simulink model "Three_phase_IM_PF_correction_Stardelta_Capacitor_Bank"  (R2024a)
settings: Solver=VariableStepAuto  StartTime=0.0  StopTime=2  RelTol=1e-3
libraries: spsRMSLib x10, spsSeriesRLCBranchLib x6, spsAsynchronousMachineSIUnitsLib x5, spsPower3phInstantaneousLib x5, spsThreePhaseVIMeasurementLib x5, spsThreePhaseSourceLib x5, spsThreePhaseSeriesRLCLoadLib x2, spspowerguiLib x1
settings Model: Creator=User  LastModifiedBy=User

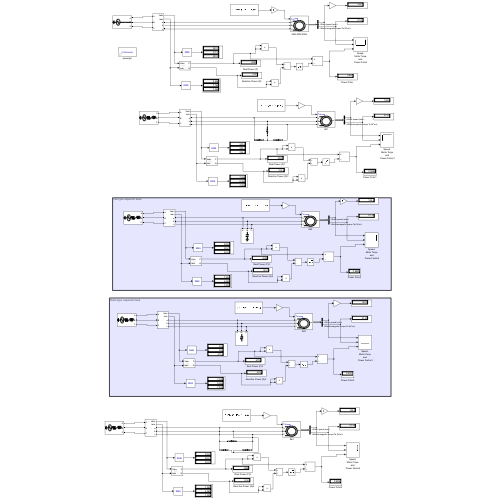
[thumbnail: Simulink's stored preview of the top-level diagram]
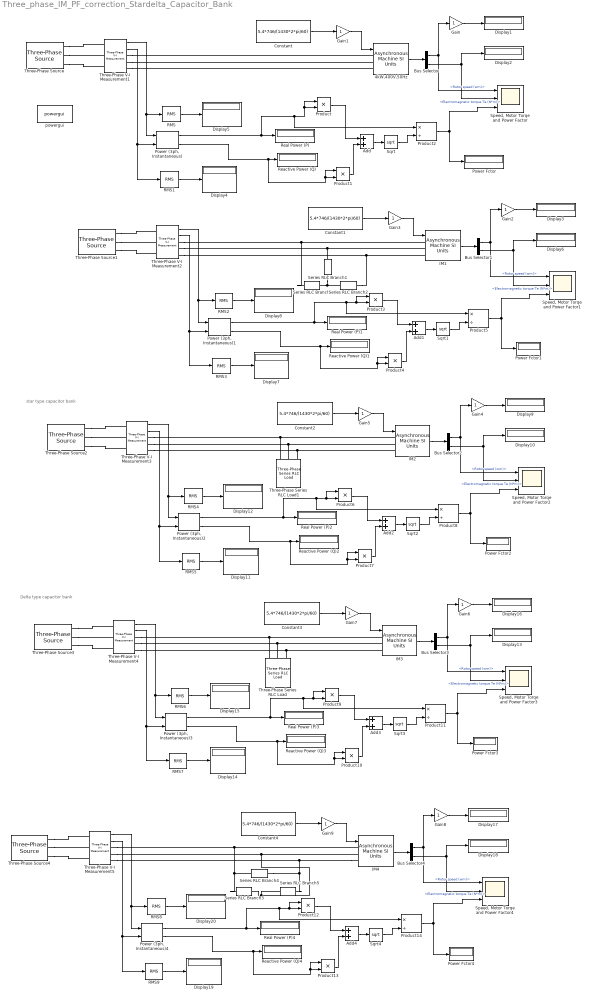
== system Three_phase_IM_PF_correction_Stardelta_Capacitor_Bank ==
  note: star type capacitor bank
  note: Delta type capacitor bank
  4kW,400V,50Hz : spsAsynchronousMachineSIUnitsLib/Asynchronous Machine SI Units  RotorType=Squirrel-cage  PresetModel="15:  5.4 HP (4KW)   400 V  50Hz 1430 RPM"  MechanicalLoad=Torque Tm  ShowDetailedParameters=on  ReferenceFrame=Rotor  Units=SI  MeasurementBus=off  NominalParameters=[4000 400 50]  VoltageRatio=1  Stator=[1.405 0.005839]  Rotor=[1.395 0.005839]  Cage1=[0.4155 0.002066]  Cage2=[0.4168 0.0003495]  Lm=0.1722  Mechanical=[0.0131 0.002985 2]  PolePairs=2  InitialConditions=[0 0 0 0 0 0 0 0]  SimulateSaturation=off  Saturation=[14.03593122, 27.81365428, 53.79336849, 72.68890987, 97.98006896, 148.6815601, 215.7428561, 302.9841135, 428.7778367 ; 230, 322, 414, 460, 506, 552, 598, 644, 690]  LoadFlowParameters=1492000  TsPowergui=0  TsBlock=-1  IterativeModel=Trapezoidal non iterative  IterativeDiscreteModel=Trapezoidal non iterative  Pmec=1.492e+006
  Add{,1..4} (5 alike) : Sum
  Bus Selector{,1..4} (5 alike) : BusSelector  OutputSignals=Mechanical.Rotor speed (wm),Mechanical.Electromagnetic torque Te (N*m)
  Constant{,1..4} (5 alike) : Constant  Value=5.4*746/(1430*2*pi/60)
  Display{1..20} (20 alike) : Display
  Gain{,1..9} (10 alike) : Gain
  IM{1..4} (4 alike) : spsAsynchronousMachineSIUnitsLib/Asynchronous Machine SI Units  RotorType=Squirrel-cage  PresetModel="15:  5.4 HP (4KW)   400 V  50Hz 1430 RPM"  MechanicalLoad=Torque Tm  ShowDetailedParameters=on  ReferenceFrame=Rotor  Units=SI  MeasurementBus=off  NominalParameters=[4000 400 50]  VoltageRatio=1  Stator=[1.405 0.005839]  Rotor=[1.395 0.005839]  Cage1=[0.4155 0.002066]  Cage2=[0.4168 0.0003495]  Lm=0.1722  Mechanical=[0.0131 0.002985 2]  PolePairs=2  InitialConditions=[0 0 0 0 0 0 0 0]  SimulateSaturation=off  Saturation=[14.03593122, 27.81365428, 53.79336849, 72.68890987, 97.98006896, 148.6815601, 215.7428561, 302.9841135, 428.7778367 ; 230, 322, 414, 460, 506, 552, 598, 644, 690]  LoadFlowParameters=1492000  TsPowergui=0  TsBlock=-1  IterativeModel=Trapezoidal non iterative  IterativeDiscreteModel=Trapezoidal non iterative  Pmec=1.492e+006
  Power (3ph, Instantaneous){,1..4} (5 alike) : spsPower3phInstantaneousLib/Power (3ph, Instantaneous)
  Power Fctor{,1..4} (5 alike) : Display
  Product{,1,3..4,6..7,9..10,12..13} (10 alike) : Product
  Product{2,5,8,11,14} (5 alike) : Product  Inputs=*/
  RMS{,1..9} (10 alike) : spsRMSLib/RMS  TrueRMS=on  Freq=60  RMSInit=120  Ts=0
  Reactive Power (Q){,1..4} (5 alike) : Display
  Real Power (P){,1..4} (5 alike) : Display
  Series RLC Branch : spsSeriesRLCBranchLib/Series RLC Branch  LConnTagsString=__new0  RConnTagsString=__new0  BranchType=C  Resistance=1  Inductance=1e-3  SetiL0=off  InitialCurrent=0  Capacitance=60.924e-6  Setx0=off  InitialVoltage=0  Measurements=None
  Series RLC Branch1 : spsSeriesRLCBranchLib/Series RLC Branch  LConnTagsString=__new0  RConnTagsString=__new0  BranchType=C  Resistance=1  Inductance=1e-3  SetiL0=off  InitialCurrent=0  Capacitance=60.924e-6  Setx0=off  InitialVoltage=0  Measurements=None
  Series RLC Branch2 : spsSeriesRLCBranchLib/Series RLC Branch  LConnTagsString=__new0  RConnTagsString=__new0  BranchType=C  Resistance=1  Inductance=1e-3  SetiL0=off  InitialCurrent=0  Capacitance=60.924e-6  Setx0=off  InitialVoltage=0  Measurements=None
  Series RLC Branch3 : spsSeriesRLCBranchLib/Series RLC Branch  LConnTagsString=__new0  RConnTagsString=__new0  BranchType=C  Resistance=1  Inductance=1e-3  SetiL0=off  InitialCurrent=0  Capacitance=20.308e-6  Setx0=off  InitialVoltage=0  Measurements=None
  Series RLC Branch4 : spsSeriesRLCBranchLib/Series RLC Branch  LConnTagsString=__new0  RConnTagsString=__new0  BranchType=C  Resistance=1  Inductance=1e-3  SetiL0=off  InitialCurrent=0  Capacitance=20.308e-6  Setx0=off  InitialVoltage=0  Measurements=None
  Series RLC Branch5 : spsSeriesRLCBranchLib/Series RLC Branch  LConnTagsString=__new0  RConnTagsString=__new0  BranchType=C  Resistance=1  Inductance=1e-3  SetiL0=off  InitialCurrent=0  Capacitance=20.308e-6  Setx0=off  InitialVoltage=0  Measurements=None
  Speed, Motor Torqe and Power Factor{,1..4} (5 alike) : Scope  NumInputPorts=3
  Sqrt{,1..4} (5 alike) : Sqrt
  Three-Phase Series RLC Load : spsThreePhaseSeriesRLCLoadLib/Three-Phase Series RLC Load  LConnTagsString=A|B|C  Configuration=Delta  NominalVoltage=400  Vabc=[1e3 1e3 1e3]  Vabcp=[1e3 1e3 1e3]  NominalFrequency=50  UnbalancedPower=off  ActivePower=0  InductivePower=0  CapacitivePower=3062.5  Pabc=[10e3 9e3 11e3]  QLabc=[100 90 110]  QCabc=[100 90 110]  Pabcp=[10e3 9e3 11e3]  QLabcp=[100 90 110]  QCabcp=[100 90 110]  Measurements=None  LoadType=constant Z
  Three-Phase Series RLC Load1 : spsThreePhaseSeriesRLCLoadLib/Three-Phase Series RLC Load  LConnTagsString=A|B|C  Configuration=Y (grounded)  NominalVoltage=400  Vabc=[1e3 1e3 1e3]  Vabcp=[1e3 1e3 1e3]  NominalFrequency=50  UnbalancedPower=off  ActivePower=0  InductivePower=0  CapacitivePower=3062.5  Pabc=[10e3 9e3 11e3]  QLabc=[100 90 110]  QCabc=[100 90 110]  Pabcp=[10e3 9e3 11e3]  QLabcp=[100 90 110]  QCabcp=[100 90 110]  Measurements=None  LoadType=constant Z
  Three-Phase V-I Measurement{1..3,5} (4 alike) : spsThreePhaseVIMeasurementLib/Three-Phase V-I Measurement  VoltageMeasurement=phase-to-ground  SetLabelV=off  LabelV=Vabc  Vpu=off  VpuLL=off  CurrentMeasurement=yes  SetLabelI=off  LabelI=Iabc  Ipu=off  Pbase=100e6  Vbase=500e3  OutputType=Complex  PhasorSimulation=off  PSBequivalent=0
  Three-Phase V-I Measurement4 : spsThreePhaseVIMeasurementLib/Three-Phase V-I Measurement  VoltageMeasurement=phase-to-phase  SetLabelV=off  LabelV=Vabc  Vpu=off  VpuLL=off  CurrentMeasurement=yes  SetLabelI=off  LabelI=Iabc  Ipu=off  Pbase=100e6  Vbase=500e3  OutputType=Complex  PhasorSimulation=off  PSBequivalent=0
  Three-Phase Source : spsThreePhaseSourceLib/Three-Phase Source  InternalConnection=Yg  VoltagePhases=off  Voltage=400  PhaseAngle=0  Voltage_phases=[25e3 25e3 25e3]/sqrt(3)  PhaseAngles_phases=[0 -120 +120]  Frequency=50  NonIdealSource=off  SpecifyImpedance=off  Resistance=0.8929  Inductance=16.58e-3  ShortCircuitLevel=100e6  BaseVoltage=400  XRratio=7  BusType=swing  Pref=10e3  Qref=0  Prefabc=[10e3, 10e3, 10e3]  Qrefabc=[0, 0, 0]  Qmin=-inf  Qmax=inf
  Three-Phase Source{1..4} (4 alike) : spsThreePhaseSourceLib/Three-Phase Source  InternalConnection=Yg  VoltagePhases=off  Voltage=400  PhaseAngle=0  Voltage_phases=[25e3 25e3 25e3]/sqrt(3)  PhaseAngles_phases=[0 -120 +120]  Frequency=50  NonIdealSource=on  SpecifyImpedance=off  Resistance=0.8929  Inductance=16.58e-3  ShortCircuitLevel=100e6  BaseVoltage=400  XRratio=7  BusType=swing  Pref=10e3  Qref=0  Prefabc=[10e3, 10e3, 10e3]  Qrefabc=[0, 0, 0]  Qmin=-inf  Qmax=inf
  powergui : spspowerguiLib/powergui  Priority=1  SimulationMode=Continuous  SampleTime=50e-6  frequency=60  Iterations=50  frequencyindice=50  Pbase=100e6  ErrMax=1e-4  UnitsV=kV  UnitsW=MW  buscounter=0  FunctionMessages=off  echomessages=off  EnableUseOfTLC=off  CurrentSourceSwitches=off  DisableSnubberDevices=off  DisableRonSwitches=off  DisableVfSwitches=off  DisplayEquations=off  AutomaticDiscreteSolvers=off  SolverType=Tustin/Backward Euler (TBE)  Interpol=off  ExternalGateDelay=off  methode=off  Ts=100  x0status=blocks  SPID=on  SwTol=0  HookPort=off  NonlinearTolerance=1e-4  nMaxIteration=100  ContinueOnMaxIteration=off  RestoreLinks=warning  ResistiveCurrentMeasurement=off  Frange=[0:2:500]  Ylog=off  Xlog=on  ShowGrid=off  save=off  variable=ZData  structure=0  ZoomFFT=off  StartTime=0.0  cycles=1  DisplayStyle=1  fundamental=60  FreqAxis=off  MaxFrequency=1000  frequencyindicesteady=1  RmsSteady=1  display=off
  wires:
  RMS1/1 -> Display4/1
  Product1/1 -> Add/2
  Gain/1 -> Display1/1
  "Power (3ph, Instantaneous)"/2 -> Product1/2, Product1/1, Reactive Power (Q)/1
  Add/1 -> Sqrt/1
  RMS/1 -> Display5/1
  Three-Phase V-I Measurement1/2 -> "Power (3ph, Instantaneous)"/2, RMS1/1
  Bus Selector/2 -> "Speed, Motor Torqe and Power Factor"/2, Display2/1  "<Electromagnetic torque Te (N*m)>"
  Product2/1 -> "Speed, Motor Torqe and Power Factor"/3, Power Fctor/1
  Product/1 -> Add/1
  Three-Phase V-I Measurement1/1 -> "Power (3ph, Instantaneous)"/1, RMS/1
  Bus Selector/1 -> "Speed, Motor Torqe and Power Factor"/1, Gain/1  "<Rotor speed (wm)>"
  "Power (3ph, Instantaneous)"/1 -> Product2/1, Product/2, Product/1, Real Power (P)/1
  Sqrt/1 -> Product2/2
  4kW,400V,50Hz/1 -> Bus Selector/1
  Constant/1 -> Gain1/1
  Gain1/1 -> 4kW,400V,50Hz/1
  Sqrt1/1 -> Product5/2
  Three-Phase V-I Measurement2/1 -> "Power (3ph, Instantaneous)1"/1, RMS2/1
  Bus Selector1/1 -> "Speed, Motor Torqe and Power Factor1"/1, Gain2/1  "<Rotor speed (wm)>"
  "Power (3ph, Instantaneous)1"/1 -> Product5/1, Product3/2, Product3/1, Real Power (P)1/1
  Product3/1 -> Add1/1
  Gain3/1 -> IM1/1
  Three-Phase V-I Measurement2/2 -> "Power (3ph, Instantaneous)1"/2, RMS3/1
  "Power (3ph, Instantaneous)1"/2 -> Product4/2, Product4/1, Reactive Power (Q)1/1
  Add1/1 -> Sqrt1/1
  Bus Selector1/2 -> "Speed, Motor Torqe and Power Factor1"/2, Display6/1  "<Electromagnetic torque Te (N*m)>"
  IM1/1 -> Bus Selector1/1
  Constant1/1 -> Gain3/1
  Product5/1 -> "Speed, Motor Torqe and Power Factor1"/3, Power Fctor1/1
  Gain2/1 -> Display3/1
  Product4/1 -> Add1/2
  RMS3/1 -> Display7/1
  RMS2/1 -> Display8/1
  "Power (3ph, Instantaneous)2"/1 -> Product8/1, Product6/2, Product6/1, Real Power (P)2/1
  RMS4/1 -> Display12/1
  Add2/1 -> Sqrt2/1
  Bus Selector2/1 -> "Speed, Motor Torqe and Power Factor2"/1, Gain4/1  "<Rotor speed (wm)>"
  Gain4/1 -> Display9/1
  Bus Selector2/2 -> "Speed, Motor Torqe and Power Factor2"/2, Display10/1  "<Electromagnetic torque Te (N*m)>"
  Product7/1 -> Add2/2
  Product8/1 -> "Speed, Motor Torqe and Power Factor2"/3, Power Fctor2/1
  Sqrt2/1 -> Product8/2
  Constant2/1 -> Gain5/1
  Gain5/1 -> IM2/1
  Product6/1 -> Add2/1
  "Power (3ph, Instantaneous)2"/2 -> Product7/2, Product7/1, Reactive Power (Q)2/1
  Three-Phase V-I Measurement3/1 -> "Power (3ph, Instantaneous)2"/1, RMS4/1
  Three-Phase V-I Measurement3/2 -> "Power (3ph, Instantaneous)2"/2, RMS5/1
  IM2/1 -> Bus Selector2/1
  RMS5/1 -> Display11/1
  IM3/1 -> Bus Selector3/1
  "Power (3ph, Instantaneous)3"/2 -> Product10/2, Product10/1, Reactive Power (Q)3/1
  Three-Phase V-I Measurement4/1 -> "Power (3ph, Instantaneous)3"/1, RMS6/1
  Product9/1 -> Add3/1
  Sqrt3/1 -> Product11/2
  Product11/1 -> "Speed, Motor Torqe and Power Factor3"/3, Power Fctor3/1
  Gain7/1 -> IM3/1
  Constant3/1 -> Gain7/1
  Product10/1 -> Add3/2
  RMS7/1 -> Display14/1
  Bus Selector3/1 -> "Speed, Motor Torqe and Power Factor3"/1, Gain6/1  "<Rotor speed (wm)>"
  "Power (3ph, Instantaneous)3"/1 -> Product11/1, Product9/2, Product9/1, Real Power (P)3/1
  Three-Phase V-I Measurement4/2 -> "Power (3ph, Instantaneous)3"/2, RMS7/1
  Gain6/1 -> Display16/1
  Bus Selector3/2 -> "Speed, Motor Torqe and Power Factor3"/2, Display13/1  "<Electromagnetic torque Te (N*m)>"
  RMS6/1 -> Display15/1
  Add3/1 -> Sqrt3/1
  "Power (3ph, Instantaneous)4"/1 -> Product14/1, Product12/2, Product12/1, Real Power (P)4/1
  RMS8/1 -> Display20/1
  Add4/1 -> Sqrt4/1
  Bus Selector4/1 -> "Speed, Motor Torqe and Power Factor4"/1, Gain8/1  "<Rotor speed (wm)>"
  Gain8/1 -> Display17/1
  Bus Selector4/2 -> "Speed, Motor Torqe and Power Factor4"/2, Display18/1  "<Electromagnetic torque Te (N*m)>"
  Product13/1 -> Add4/2
  Product14/1 -> "Speed, Motor Torqe and Power Factor4"/3, Power Fctor4/1
  Sqrt4/1 -> Product14/2
  Constant4/1 -> Gain9/1
  Gain9/1 -> IM4/1
  Product12/1 -> Add4/1
  "Power (3ph, Instantaneous)4"/2 -> Product13/2, Product13/1, Reactive Power (Q)4/1
  Three-Phase V-I Measurement5/1 -> "Power (3ph, Instantaneous)4"/1, RMS8/1
  Three-Phase V-I Measurement5/2 -> "Power (3ph, Instantaneous)4"/2, RMS9/1
  IM4/1 -> Bus Selector4/1
  RMS9/1 -> Display19/1
  connections:
  Three-Phase V-I Measurement1/RConn2 -- 4kW,400V,50Hz/LConn2
  Three-Phase V-I Measurement1/RConn1 -- 4kW,400V,50Hz/LConn1
  Three-Phase V-I Measurement1/RConn3 -- 4kW,400V,50Hz/LConn3
  Three-Phase Source/RConn1 -- Three-Phase V-I Measurement1/LConn1
  Three-Phase Source/RConn2 -- Three-Phase V-I Measurement1/LConn2
  Three-Phase Source/RConn3 -- Three-Phase V-I Measurement1/LConn3
  Three-Phase V-I Measurement2/RConn2 -- Series RLC Branch1/LConn1 -- IM1/LConn2
  Three-Phase V-I Measurement2/RConn3 -- Series RLC Branch2/RConn1 -- IM1/LConn3
  Three-Phase V-I Measurement2/RConn1 -- Series RLC Branch/LConn1 -- IM1/LConn1
  Three-Phase Source1/RConn3 -- Three-Phase V-I Measurement2/LConn3
  Three-Phase Source1/RConn1 -- Three-Phase V-I Measurement2/LConn1
  Three-Phase Source1/RConn2 -- Three-Phase V-I Measurement2/LConn2
  Series RLC Branch/RConn1 -- Series RLC Branch1/RConn1 -- Series RLC Branch2/LConn1
  Three-Phase V-I Measurement3/RConn3 -- Three-Phase Series RLC Load1/LConn3 -- IM2/LConn3
  Three-Phase V-I Measurement3/RConn1 -- Three-Phase Series RLC Load1/LConn1 -- IM2/LConn1
  Three-Phase Source2/RConn1 -- Three-Phase V-I Measurement3/LConn1
  Three-Phase Source2/RConn3 -- Three-Phase V-I Measurement3/LConn3
  Three-Phase Source2/RConn2 -- Three-Phase V-I Measurement3/LConn2
  Three-Phase V-I Measurement4/RConn1 -- Three-Phase Series RLC Load/LConn1 -- IM3/LConn1
  Three-Phase Source3/RConn3 -- Three-Phase V-I Measurement4/LConn3
  Three-Phase Source3/RConn1 -- Three-Phase V-I Measurement4/LConn1
  Three-Phase Source3/RConn2 -- Three-Phase V-I Measurement4/LConn2
  Three-Phase V-I Measurement4/RConn2 -- Three-Phase Series RLC Load/LConn2 -- IM3/LConn2
  Three-Phase V-I Measurement4/RConn3 -- Three-Phase Series RLC Load/LConn3 -- IM3/LConn3
  Three-Phase V-I Measurement3/RConn2 -- Three-Phase Series RLC Load1/LConn2 -- IM2/LConn2
  IM4/LConn3 -- Series RLC Branch4/LConn1 -- Series RLC Branch5/RConn1 -- Three-Phase V-I Measurement5/RConn3
  Three-Phase V-I Measurement5/RConn1 -- Series RLC Branch4/RConn1 -- Series RLC Branch3/LConn1 -- IM4/LConn1
  Three-Phase V-I Measurement5/RConn2 -- Series RLC Branch5/LConn1 -- Series RLC Branch3/RConn1 -- IM4/LConn2
  Three-Phase Source4/RConn3 -- Three-Phase V-I Measurement5/LConn3
  Three-Phase Source4/RConn1 -- Three-Phase V-I Measurement5/LConn1
  Three-Phase Source4/RConn2 -- Three-Phase V-I Measurement5/LConn2
